simulink model "EKF_pendulum"  (R2019b)
settings: Solver=FixedStepAuto  StartTime=0.0  StopTime=10.0  FixedStep=sim_freq  RelTol=1e-3
values from neighbouring files (symbols this model uses):
  b = 0.1    [myStateTransitionFcn.m]    (also in pendulum_EKF.m = 0.5; random_walk_pendulum_EKF.m)
  g = 9.81    [myStateTransitionFcn.m]    (also in pendulum_EKF.m; random_walk_pendulum_EKF.m)
  I = 0.1    [myStateTransitionFcn.m]    (also in pendulum_EKF.m = 2; random_walk_pendulum_EKF.m)
  L = 0.5    [myStateTransitionFcn.m]    (also in pendulum_EKF.m = 1; random_walk_pendulum_EKF.m)
  m = 1    [myStateTransitionFcn.m]    (also in pendulum_EKF.m = 2; random_walk_pendulum_EKF.m)
  meas_theta_dot_var = 0.0001    [pendulum_EKF.m]    (also in random_walk_pendulum_EKF.m = 1e-06)
  meas_theta_var = 0.0001    [pendulum_EKF.m]    (also in random_walk_pendulum_EKF.m = 1e-06)
  Pk_init = zeros(2)    [pendulum_EKF.m]    (also in random_walk_pendulum_EKF.m = zeros(3))
  Qk = C22'*C12    [pendulum_EKF.m]    (also in random_walk_pendulum_EKF.m; symbolic_pendulum_ekf.m = eye(2)*[process_theta_variance;process_theta_dot_variance]*T; symbolic_pendulum_random_walk_ekf.m = eye(2)*[process_theta_variance;process_theta_dot_variance]*T)
  Rk = [meas_theta_var 0; 0 meas_theta_dot_var]    [pendulum_EKF.m]    (also in random_walk_pendulum_EKF.m = [meas_theta_var 0 ; 0 meas_theta_dot_var])
  Ts = 0.004    [pendulum_EKF.m]    (also in random_walk_pendulum_EKF.m; symbolic_pendulum_ekf.m; symbolic_pendulum_random_walk_ekf.m)
  X_hat_init = [0;0]    [pendulum_EKF.m]    (also in random_walk_pendulum_EKF.m = [0;0;0])
libraries: simulink x1
settings Model: Creator=henry  LastModifiedBy=henry

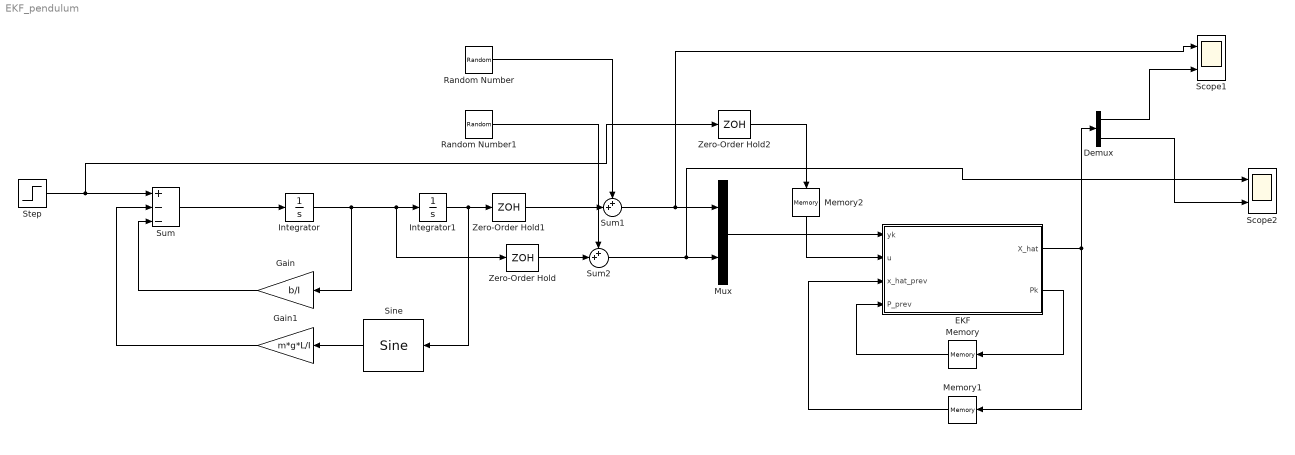
== system EKF_pendulum ==
  Demux : Demux  Outputs=2
  EKF : MATLAB Function  TreatAsAtomicUnit=on
  Gain : Gain  Gain=b/I
  Gain1 : Gain  Gain=m*g*L/I
  Integrator : Integrator
  Integrator1 : Integrator
  Memory : Memory  InitialCondition=Pk_init
  Memory1 : Memory  InitialCondition=X_hat_init
  Memory2 : Memory
  Mux : Mux  Inputs=2
  Random Number : RandomNumber  Variance=meas_theta_var  Seed=1  SampleTime=Ts
  Random Number1 : RandomNumber  Variance=meas_theta_dot_var  Seed=2  SampleTime=Ts
  Scope1 : Scope  NumInputPorts=2
  Scope2 : Scope  NumInputPorts=2
  Sine : simulink/Lookup Tables/Sine  Formula=sin(2*pi*u)  NumDataPoints=(2^5)+1  OutputWordLength=16  InternalRulePriority=Precision
      settings: SourceProductName=Simulink
  Step : Step  Time=2  After=5  SampleTime=0
  Sum : Sum  Inputs=+--
  Sum1 : Sum  Inputs=++|
  Sum2 : Sum  Inputs=++|
  Zero-Order Hold : ZeroOrderHold  SampleTime=Ts
  Zero-Order Hold1 : ZeroOrderHold  SampleTime=Ts
  Zero-Order Hold2 : ZeroOrderHold  SampleTime=Ts
  wires:
  Integrator/1 -> Gain/1, Zero-Order Hold/1, Integrator1/1
  Sum/1 -> Integrator/1
  Gain/1 -> Sum/3
  Gain1/1 -> Sum/2
  Random Number/1 -> Sum1/1
  Mux/1 -> EKF/1(yk)
  Sum2/1 -> Scope2/1, Mux/2
  Sum1/1 -> Scope1/1, Mux/1
  EKF/2(Pk) -> Memory/1
  Memory/1 -> EKF/4(P_prev)
  EKF/1(X_hat) -> Memory1/1, Demux/1
  Memory1/1 -> EKF/3(x_hat_prev)
  Sine/1 -> Gain1/1
  Random Number1/1 -> Sum2/1
  Memory2/1 -> EKF/2(u)
  Zero-Order Hold/1 -> Sum2/2
  Zero-Order Hold1/1 -> Sum1/2
  Step/1 -> Zero-Order Hold2/1, Sum/1
  Integrator1/1 -> Zero-Order Hold1/1, Sine/1
  Demux/1 -> Scope1/2
  Demux/2 -> Scope2/2
  Zero-Order Hold2/1 -> Memory2/1

== matlab function EKF_pendulum/EKF ==
  data: yk input size=[2 1]; u input; X_hat output size=[2 1]; x_hat_prev input size=[2 1]; P_prev input size=[2 2]; Pk output size=[2 2]; m parameter; g parameter; L parameter; I parameter; b parameter; Qk parameter size=[2 2]; Rk parameter size=[2 2]
function [X_hat,Pk]= fcn(yk,u,x_hat_prev,P_prev,m, g, L, I, b, Qk, Rk)


F1 = @(x,u) x(2);
F2 = @(x,u) u/I - (m*g*L/I)*sin( x(1) ) - x(2)*b/I;
H1 = @(x) x(1);
H2 = @(x) x(2);

Fk = @(x,u) [1, 1/250; -(L*g*m*cos(x(1)))/(250*I), 1 - b/(250*I)];

%% update Qk


%% Control Update
Pk_ =  Fk(x_hat_prev,u) * P_prev * transpose( Fk(x_hat_prev,u) ) + Qk;
Xk_ = x_hat_prev + [ F1(x_hat_prev,u) ; F2(x_hat_prev,u) ]*1/250; 

Hk = [1 0 ;0 1];

%% Measurement Update
Lk = Pk_*transpose(Hk)*inv(Hk*Pk_*transpose(Hk) + Rk);
Pk = (eye(2) - Lk*Hk)*Pk_;
X_hat = Xk_ + Lk*(yk - [ H1(Xk_);H2(Xk_)]);
